simulink model "BikeModelDynWheels"  (R2017b)
settings: Solver=VariableStepAuto  StartTime=0.0  StopTime=10.0  RelTol=1e-3
undefined symbols (not defined in the file): b_contact, C_F_alpha, C_F_kappa, Cylinder, Dphi0, Dpsi0, epsilon, g, k_contact, lengthFF, lengthRF, lengthRW, locY, locZ, massRW, mB, mH, Parts_Lib, radiusRW, sigma, X, xPla, Y, yPla, Z, zPla
libraries: sm_lib x24, nesl_utility x18, vrlib x8, dspsrcs4 x1
(part 1 of 2)
settings Model: Creator=r_ahmed_afzal  LastModifiedBy=r_ahmed_afzal

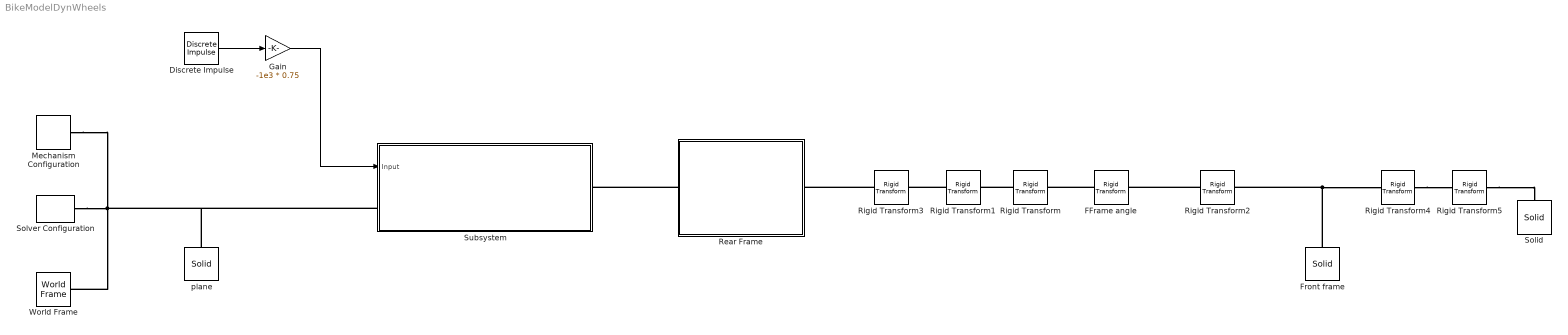
== system BikeModelDynWheels ==
  Discrete Impulse : dspsrcs4/Discrete  Impulse  Delay=0  SampleTime=1e-2  FrameSample=1  OutputFrames=off  dataType=double  isSigned=on  wordLen=16  udDataType=sfix(16)  fracBitsMode=Best precision  numFracBits=15  OutDataTypeStr=double  LastOutDataTypeStr=double
  FFrame angle : sm_lib/Frames and Transforms/Rigid Transform  TranslationMethod=None  TranslationStandardOffset=0  TranslationLengthUnit=m  TranslationStandardAxis=+Z  TranslationCartesianOffset=[0 0 0]  TranslationROffset=0  TranslationROffsetUnits=m  TranslationZOffset=0  TranslationZOffsetUnits=m  TranslationThetaOffset=0  TranslationThetaOffsetUnits=deg  RotationMethod=StandardAxis  RotationAngleUnits=rad  RotationStandardAxis=+X  RotationAngle=angleFF  RotationArbitraryAxis=[0 0 1]  FollAlignAxisA=+X  BaseAlignAxisA=+Y  FollAlignAxisB=+Y  BaseAlignAxisB=+Z  RotationSequenceAxes=FollowerAxes  RotationSequence=XYX  RotationSequenceAngles=[0 0 0]  RotationSequenceAnglesUnits=deg  RotationMatrix=[1 0 0; 0 1 0; 0 0 1]
  Front frame : sm_lib/Body Elements/Solid  InertiaType=Custom  Mass=mH  MassUnits=kg  CenterOfMass=[0 0 0]  CenterOfMassUnits=m  MomentsOfInertia=[1 1 1]  MomentsOfInertiaUnits=kg*m^2  ProductsOfInertia=[1 1 1]  ProductsOfInertiaUnits=kg*m^2  DensityBased=on  Density=1000  DensityUnits=kg/m^3  DoExposeReferenceFrame=on  SerializedFrames=<Frames/>  GraphicType=FromGeometry  MarkerShape=Sphere  MarkerSize=10  GraphicVisPropType=SimpleVisualProperties  GraphicDiffuseColor=[0.2 0.6 0.0]  GraphicSpecularColor=[0.5 0.5 0.5 1.0]  GraphicAmbientColor=[0.15 0.15 0.15 1.0]  GraphicEmissiveColor=[0.0 0.0 0.0 1.0]  GraphicShininess=75  GraphicOpacity=1.0  GeometryShape=Cylinder  RectangleSize=[1 1]  RectangleSizeUnits=m  BrickDimensions=[1 1 1]  BrickDimensionUnits=m  CylinderRadius=cylFF  CylinderRadiusUnits=m  CylinderLength=lengthFF  CylinderLengthUnits=m  SphereRadius=1  SphereRadiusUnits=m  EllipsoidRadii=[1 1 1]  EllipsoidRadiiUnits=m  ExtrusionCrossSection=[1 1; -1 1; -1 -1; 1 -1]  ExtrusionCrossSectionUnits=m  ExtrusionLength=1  ExtrusionLengthUnits=m  PolygonNumSides=3  PolygonOuterRadius=1  PolygonOuterRadiusUnits=m  ExtGeomFileType=STEP  ExtGeomFileUnits=m  RevolutionCrossSection=[1 1; 1 -1; 2 -1; 2 1]  RevolutionCrossSectionUnits=m  RevolutionExtent=Full  RevolutionAngle=180  RevolutionAngleUnits=deg
  Gain : Gain  Gain=-1e3 * 0.75
  Mechanism Configuration : sm_lib/Utilities/Mechanism Configuration  UniformGravity=Constant  GravityVector=[0 0 -g]  GravityUnits=m/s^2  LinearizationDelta=0.001
  Rear Frame : Subsystem
  Rigid Transform : sm_lib/Frames and Transforms/Rigid Transform  TranslationMethod=None  TranslationStandardOffset=0  TranslationLengthUnit=m  TranslationStandardAxis=+Z  TranslationCartesianOffset=[0 0 0]  TranslationROffset=0  TranslationROffsetUnits=m  TranslationZOffset=0  TranslationZOffsetUnits=m  TranslationThetaOffset=0  TranslationThetaOffsetUnits=deg  RotationMethod=None  RotationAngleUnits=deg  RotationStandardAxis=+Z  RotationAngle=0.0  RotationArbitraryAxis=[0 0 1]  FollAlignAxisA=+X  BaseAlignAxisA=+Y  FollAlignAxisB=+Y  BaseAlignAxisB=+Z  RotationSequenceAxes=FollowerAxes  RotationSequence=XYX  RotationSequenceAngles=[0 0 0]  RotationSequenceAnglesUnits=deg  RotationMatrix=[1 0 0; 0 1 0; 0 0 1]
  Rigid Transform1 : sm_lib/Frames and Transforms/Rigid Transform  TranslationMethod=None  TranslationStandardOffset=0  TranslationLengthUnit=m  TranslationStandardAxis=+Z  TranslationCartesianOffset=[0 0 0]  TranslationROffset=0  TranslationROffsetUnits=m  TranslationZOffset=0  TranslationZOffsetUnits=m  TranslationThetaOffset=0  TranslationThetaOffsetUnits=deg  RotationMethod=StandardAxis  RotationAngleUnits=rad  RotationStandardAxis=+X  RotationAngle=angleRF  RotationArbitraryAxis=[0 0 1]  FollAlignAxisA=+X  BaseAlignAxisA=+Y  FollAlignAxisB=+Y  BaseAlignAxisB=+Z  RotationSequenceAxes=FollowerAxes  RotationSequence=XYX  RotationSequenceAngles=[0 0 0]  RotationSequenceAnglesUnits=deg  RotationMatrix=[1 0 0; 0 1 0; 0 0 1]
  Rigid Transform2 : sm_lib/Frames and Transforms/Rigid Transform  TranslationMethod=StandardAxis  TranslationStandardOffset=lengthFF/2  TranslationLengthUnit=m  TranslationStandardAxis=+Z  TranslationCartesianOffset=[0 0 0]  TranslationROffset=0  TranslationROffsetUnits=m  TranslationZOffset=0  TranslationZOffsetUnits=m  TranslationThetaOffset=0  TranslationThetaOffsetUnits=deg  RotationMethod=None  RotationAngleUnits=deg  RotationStandardAxis=+Z  RotationAngle=0.0  RotationArbitraryAxis=[0 0 1]  FollAlignAxisA=+X  BaseAlignAxisA=+Y  FollAlignAxisB=+Y  BaseAlignAxisB=+Z  RotationSequenceAxes=FollowerAxes  RotationSequence=XYX  RotationSequenceAngles=[0 0 0]  RotationSequenceAnglesUnits=deg  RotationMatrix=[1 0 0; 0 1 0; 0 0 1]
  Rigid Transform3 : sm_lib/Frames and Transforms/Rigid Transform  TranslationMethod=StandardAxis  TranslationStandardOffset=lengthRF/2  TranslationLengthUnit=m  TranslationStandardAxis=+Z  TranslationCartesianOffset=[0 0 0]  TranslationROffset=0  TranslationROffsetUnits=m  TranslationZOffset=0  TranslationZOffsetUnits=m  TranslationThetaOffset=0  TranslationThetaOffsetUnits=deg  RotationMethod=None  RotationAngleUnits=deg  RotationStandardAxis=+Z  RotationAngle=0.0  RotationArbitraryAxis=[0 0 1]  FollAlignAxisA=+X  BaseAlignAxisA=+Y  FollAlignAxisB=+Y  BaseAlignAxisB=+Z  RotationSequenceAxes=FollowerAxes  RotationSequence=XYX  RotationSequenceAngles=[0 0 0]  RotationSequenceAnglesUnits=deg  RotationMatrix=[1 0 0; 0 1 0; 0 0 1]
  Rigid Transform4 : sm_lib/Frames and Transforms/Rigid Transform  TranslationMethod=StandardAxis  TranslationStandardOffset=lengthFF/2  TranslationLengthUnit=m  TranslationStandardAxis=+Z  TranslationCartesianOffset=[0 0 0]  TranslationROffset=0  TranslationROffsetUnits=m  TranslationZOffset=0  TranslationZOffsetUnits=m  TranslationThetaOffset=0  TranslationThetaOffsetUnits=deg  RotationMethod=StandardAxis  RotationAngleUnits=rad  RotationStandardAxis=-X  RotationAngle=angleFF  RotationArbitraryAxis=[0 0 1]  FollAlignAxisA=+X  BaseAlignAxisA=+Y  FollAlignAxisB=+Y  BaseAlignAxisB=+Z  RotationSequenceAxes=FollowerAxes  RotationSequence=XYX  RotationSequenceAngles=[0 0 0]  RotationSequenceAnglesUnits=deg  RotationMatrix=[1 0 0; 0 1 0; 0 0 1]
  Rigid Transform5 : sm_lib/Frames and Transforms/Rigid Transform  TranslationMethod=None  TranslationStandardOffset=0  TranslationLengthUnit=m  TranslationStandardAxis=+Z  TranslationCartesianOffset=[0 0 0]  TranslationROffset=0  TranslationROffsetUnits=m  TranslationZOffset=0  TranslationZOffsetUnits=m  TranslationThetaOffset=0  TranslationThetaOffsetUnits=deg  RotationMethod=AlignedAxes  RotationAngleUnits=deg  RotationStandardAxis=+Z  RotationAngle=0.0  RotationArbitraryAxis=[0 0 1]  FollAlignAxisA=+X  BaseAlignAxisA=+Z  FollAlignAxisB=+Z  BaseAlignAxisB=-X  RotationSequenceAxes=FollowerAxes  RotationSequence=XYX  RotationSequenceAngles=[0 0 0]  RotationSequenceAnglesUnits=deg  RotationMatrix=[1 0 0; 0 1 0; 0 0 1]
  Solid : sm_lib/Body Elements/Solid  InertiaType=CalculateFromGeometry  Mass=1  MassUnits=kg  CenterOfMass=[0 0 0]  CenterOfMassUnits=m  MomentsOfInertia=[1 1 1]  MomentsOfInertiaUnits=kg*m^2  ProductsOfInertia=[1 1 1]  ProductsOfInertiaUnits=kg*m^2  DensityBased=on  Density=1000  DensityUnits=kg/m^3  DoExposeReferenceFrame=on  SerializedFrames=<Frames/>  GraphicType=FromGeometry  MarkerShape=Sphere  MarkerSize=10  GraphicVisPropType=SimpleVisualProperties  GraphicDiffuseColor=[0.5 0.5 0.5]  GraphicSpecularColor=[0.5 0.5 0.5 1.0]  GraphicAmbientColor=[0.15 0.15 0.15 1.0]  GraphicEmissiveColor=[0.0 0.0 0.0 1.0]  GraphicShininess=75  GraphicOpacity=1.0  GeometryShape=Cylinder  RectangleSize=[1 1]  RectangleSizeUnits=m  BrickDimensions=[1 1 1]  BrickDimensionUnits=m  CylinderRadius=radiusFW  CylinderRadiusUnits=m  CylinderLength=lengthFW  CylinderLengthUnits=m  SphereRadius=1  SphereRadiusUnits=m  EllipsoidRadii=[1 1 1]  EllipsoidRadiiUnits=m  ExtrusionCrossSection=[1 1; -1 1; -1 -1; 1 -1]  ExtrusionCrossSectionUnits=m  ExtrusionLength=1  ExtrusionLengthUnits=m  PolygonNumSides=3  PolygonOuterRadius=1  PolygonOuterRadiusUnits=m  ExtGeomFileType=STEP  ExtGeomFileUnits=m  RevolutionCrossSection=[1 1; 1 -1; 2 -1; 2 1]  RevolutionCrossSectionUnits=m  RevolutionExtent=Full  RevolutionAngle=180  RevolutionAngleUnits=deg
  Solver Configuration : nesl_utility/Solver Configuration  PhysicalDomain=network_engine_domain  SubClassName=solver  LeftPortType=input  RightPortType=generic  Accelerate=off  Tones=[]  Harmonics=[]  SimulateNoise=off  Profile=off  UseLocalSampling=off  EnableSwitchedLinearOptims=on  FrequencyDomain=off  UseCCode=off  RelTol=0.001  AbsTol=1e-06  MinStep=1e-09  ToWorkspace=off  RevertToSquareIcSolve=off  NumHomotopyIterations=100  PhasorMode=off  PhasorModeNumHarmonics=1  DoDC=off  ResidualTolerance=1e-09  UseLocalSolver=off  LocalSolverChoice=NE_BACKWARD_EULER_ADVANCER  LocalSolverSampleTime=0.001  DoFixedCost=off  MaxNonlinIter=3  MaxModeIter=2  LinearAlgebra=Sparse  DelaysMemoryBudget=1024  AutomaticFiltering=on  FilteringTimeConstant=0.001
  Subsystem : Subsystem
  World Frame : sm_lib/Frames and Transforms/World Frame
  plane : sm_lib/Body Elements/Solid  InertiaType=CalculateFromGeometry  Mass=1  MassUnits=kg  CenterOfMass=[0 0 0]  CenterOfMassUnits=m  MomentsOfInertia=[1 1 1]  MomentsOfInertiaUnits=kg*m^2  ProductsOfInertia=[1 1 1]  ProductsOfInertiaUnits=kg*m^2  DensityBased=on  Density=1000  DensityUnits=kg/m^3  DoExposeReferenceFrame=on  SerializedFrames=<Frames/>  GraphicType=FromGeometry  MarkerShape=Sphere  MarkerSize=10  GraphicVisPropType=SimpleVisualProperties  GraphicDiffuseColor=[0.5 0.5 0.5]  GraphicSpecularColor=[0.5 0.5 0.5 1.0]  GraphicAmbientColor=[0.15 0.15 0.15 1.0]  GraphicEmissiveColor=[0.0 0.0 0.0 1.0]  GraphicShininess=75  GraphicOpacity=0.5  GeometryShape=Brick  RectangleSize=[1 1]  RectangleSizeUnits=m  BrickDimensions=[xPla yPla zPla]  BrickDimensionUnits=m  CylinderRadius=1  CylinderRadiusUnits=m  CylinderLength=1  CylinderLengthUnits=m  SphereRadius=1  SphereRadiusUnits=m  EllipsoidRadii=[1 1 1]  EllipsoidRadiiUnits=m  ExtrusionCrossSection=[1 1; -1 1; -1 -1; 1 -1]  ExtrusionCrossSectionUnits=m  ExtrusionLength=1  ExtrusionLengthUnits=m  PolygonNumSides=3  PolygonOuterRadius=1  PolygonOuterRadiusUnits=m  ExtGeomFileType=STEP  ExtGeomFileUnits=m  RevolutionCrossSection=[1 1; 1 -1; 2 -1; 2 1]  RevolutionCrossSectionUnits=m  RevolutionExtent=Full  RevolutionAngle=180  RevolutionAngleUnits=deg
  wires:
  Discrete Impulse/1 -> Gain/1
  Gain/1 -> Subsystem/1(Input)
  connections:
  Mechanism Configuration/RConn1 -- Subsystem/LConn1 -- plane/RConn1 -- Solver Configuration/RConn1 -- World Frame/RConn1
  Rear Frame/LConn1 -- Subsystem/RConn1
  Rigid Transform3/LConn1 -- Rear Frame/RConn1
  Rigid Transform1/LConn1 -- Rigid Transform3/RConn1
  Rigid Transform/LConn1 -- Rigid Transform1/RConn1
  FFrame angle/LConn1 -- Rigid Transform/RConn1
  Rigid Transform2/LConn1 -- FFrame angle/RConn1
  Front frame/RConn1 -- Rigid Transform4/LConn1 -- Rigid Transform2/RConn1
  Rigid Transform5/RConn1 -- Solid/RConn1
  Rigid Transform4/RConn1 -- Rigid Transform5/LConn1

== system BikeModelDynWheels/Rear Frame ==
  Rframe : sm_lib/Body Elements/Solid  InertiaType=Custom  Mass=mB  MassUnits=kg  CenterOfMass=[0 locY locZ]  CenterOfMassUnits=m  MomentsOfInertia=[1 1 1]  MomentsOfInertiaUnits=kg*m^2  ProductsOfInertia=[1 1 1]  ProductsOfInertiaUnits=kg*m^2  DensityBased=on  Density=1000  DensityUnits=kg/m^3  DoExposeReferenceFrame=on  SerializedFrames=<Frames/>  GraphicType=FromGeometry  MarkerShape=Sphere  MarkerSize=10  GraphicVisPropType=SimpleVisualProperties  GraphicDiffuseColor=[0.2 0.6 0.0]  GraphicSpecularColor=[0.5 0.5 0.5 1.0]  GraphicAmbientColor=[0.15 0.15 0.15 1.0]  GraphicEmissiveColor=[0.0 0.0 0.0 1.0]  GraphicShininess=75  GraphicOpacity=1.0  GeometryShape=Cylinder  RectangleSize=[1 1]  RectangleSizeUnits=m  BrickDimensions=[1 1 1]  BrickDimensionUnits=m  CylinderRadius=cylRF  CylinderRadiusUnits=m  CylinderLength=lengthRF  CylinderLengthUnits=m  SphereRadius=1  SphereRadiusUnits=m  EllipsoidRadii=[1 1 1]  EllipsoidRadiiUnits=m  ExtrusionCrossSection=[1 1; -1 1; -1 -1; 1 -1]  ExtrusionCrossSectionUnits=m  ExtrusionLength=1  ExtrusionLengthUnits=m  PolygonNumSides=3  PolygonOuterRadius=1  PolygonOuterRadiusUnits=m  ExtGeomFileType=STEP  ExtGeomFileUnits=m  RevolutionCrossSection=[1 1; 1 -1; 2 -1; 2 1]  RevolutionCrossSectionUnits=m  RevolutionExtent=Full  RevolutionAngle=180  RevolutionAngleUnits=deg
  Rigid Transform : sm_lib/Frames and Transforms/Rigid Transform  TranslationMethod=None  TranslationStandardOffset=0  TranslationLengthUnit=m  TranslationStandardAxis=+Z  TranslationCartesianOffset=[0 0 0]  TranslationROffset=0  TranslationROffsetUnits=m  TranslationZOffset=0  TranslationZOffsetUnits=m  TranslationThetaOffset=0  TranslationThetaOffsetUnits=deg  RotationMethod=StandardAxis  RotationAngleUnits=deg  RotationStandardAxis=+Y  RotationAngle=90  RotationArbitraryAxis=[0 0 1]  FollAlignAxisA=+X  BaseAlignAxisA=+Y  FollAlignAxisB=+Y  BaseAlignAxisB=+Z  RotationSequenceAxes=FollowerAxes  RotationSequence=XYX  RotationSequenceAngles=[0 0 0]  RotationSequenceAnglesUnits=deg  RotationMatrix=[1 0 0; 0 1 0; 0 0 1]
  Rigid Transform1 : sm_lib/Frames and Transforms/Rigid Transform  TranslationMethod=None  TranslationStandardOffset=0  TranslationLengthUnit=m  TranslationStandardAxis=+Z  TranslationCartesianOffset=[0 0 0]  TranslationROffset=0  TranslationROffsetUnits=m  TranslationZOffset=0  TranslationZOffsetUnits=m  TranslationThetaOffset=0  TranslationThetaOffsetUnits=deg  RotationMethod=StandardAxis  RotationAngleUnits=rad  RotationStandardAxis=-X  RotationAngle=angleRF  RotationArbitraryAxis=[0 0 1]  FollAlignAxisA=+X  BaseAlignAxisA=+Y  FollAlignAxisB=+Y  BaseAlignAxisB=+Z  RotationSequenceAxes=FollowerAxes  RotationSequence=XYX  RotationSequenceAngles=[0 0 0]  RotationSequenceAnglesUnits=deg  RotationMatrix=[1 0 0; 0 1 0; 0 0 1]
  Rigid Transform2 : sm_lib/Frames and Transforms/Rigid Transform  TranslationMethod=StandardAxis  TranslationStandardOffset=lengthRF/2  TranslationLengthUnit=m  TranslationStandardAxis=+Z  TranslationCartesianOffset=[0 0 0]  TranslationROffset=0  TranslationROffsetUnits=m  TranslationZOffset=0  TranslationZOffsetUnits=m  TranslationThetaOffset=0  TranslationThetaOffsetUnits=deg  RotationMethod=None  RotationAngleUnits=deg  RotationStandardAxis=+Z  RotationAngle=0.0  RotationArbitraryAxis=[0 0 1]  FollAlignAxisA=+X  BaseAlignAxisA=+Y  FollAlignAxisB=+Y  BaseAlignAxisB=+Z  RotationSequenceAxes=FollowerAxes  RotationSequence=XYX  RotationSequenceAngles=[0 0 0]  RotationSequenceAnglesUnits=deg  RotationMatrix=[1 0 0; 0 1 0; 0 0 1]
  Conn1 : PMIOPort  Port=1  Side=Left
  Conn2 : PMIOPort  Port=2  Side=Right
  connections:
  Rigid Transform1/LConn1 -- Rigid Transform/RConn1
  Rframe/RConn1 -- Conn2/RConn1 -- Rigid Transform2/RConn1
  Rigid Transform/LConn1 -- Conn1/RConn1
  Rigid Transform2/LConn1 -- Rigid Transform1/RConn1

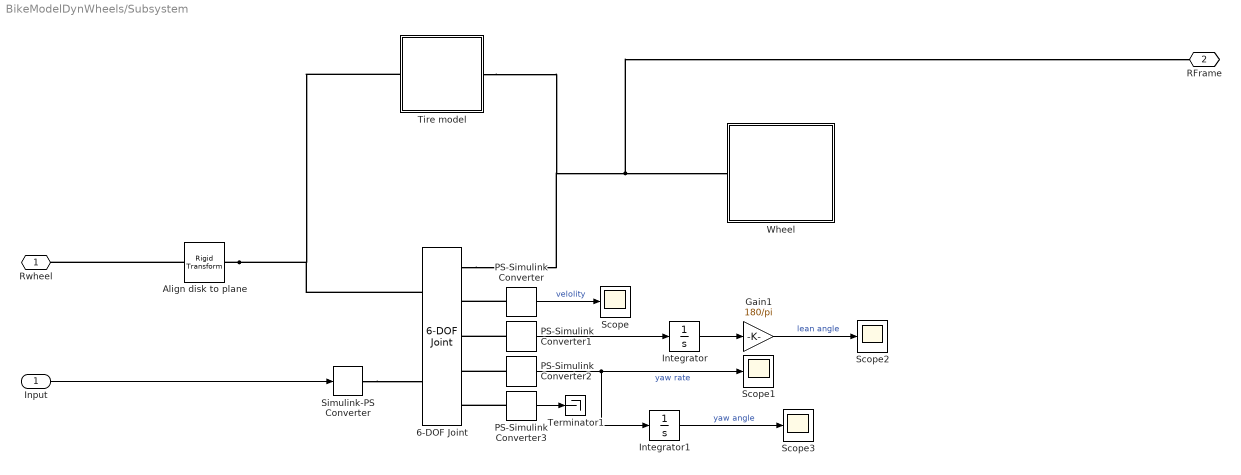
== system BikeModelDynWheels/Subsystem ==
  Input : Inport
  6-DOF Joint : sm_lib/Joints/6-DOF Joint  SenseConstraintForce=off  SenseConstraintForceX=off  SenseConstraintForceY=off  SenseConstraintForceZ=off  SenseConstraintTorque=off  SenseConstraintTorqueX=off  SenseConstraintTorqueY=off  SenseConstraintTorqueZ=off  SenseTotalForce=off  SenseTotalForceX=off  SenseTotalForceY=off  SenseTotalForceZ=off  SenseTotalTorque=off  SenseTotalTorqueX=off  SenseTotalTorqueY=off  SenseTotalTorqueZ=off  CompositeWrenchDir=FollowerOnBase  CompositeWrenchFrame=BaseFrame  PxEquilibriumPosition=0  PxEquilibriumPositionUnits=m  PxSpringStiffness=0  PxSpringStiffnessUnits=N/m  PxDampingCoefficient=0  PxDampingCoefficientUnits=N/(m/s)  PxTorqueActuationMode=NoTorque  PxMotionActuationMode=ComputedMotion  PxSensePosition=off  PxSenseVelocity=on  PxSenseAcceleration=off  PxSenseTorqueForce=off  PxPositionTargetSpecify=on  PxPositionTargetPriority=High  PxPositionTargetValue=-xPla/2 + 0.1  PxPositionTargetValueUnits=m  PxVelocityTargetSpecify=off  PxVelocityTargetPriority=High  PxVelocityTargetValue=v0  PxVelocityTargetValueUnits=m/s  PyEquilibriumPosition=0  PyEquilibriumPositionUnits=m  PySpringStiffness=0  PySpringStiffnessUnits=N/m  PyDampingCoefficient=0  PyDampingCoefficientUnits=N/(m/s)  PyTorqueActuationMode=NoTorque  PyMotionActuationMode=ComputedMotion  PySensePosition=off  PySenseVelocity=off  PySenseAcceleration=off  PySenseTorqueForce=off  PyPositionTargetSpecify=on  PyPositionTargetPriority=High  PyPositionTargetValue=radiusRW  PyPositionTargetValueUnits=m  PyVelocityTargetSpecify=off  PyVelocityTargetPriority=High  PyVelocityTargetValue=0  PyVelocityTargetValueUnits=m/s  PzEquilibriumPosition=0  PzEquilibriumPositionUnits=m  PzSpringStiffness=0  PzSpringStiffnessUnits=N/m  PzDampingCoefficient=0  PzDampingCoefficientUnits=N/(m/s)  PzTorqueActuationMode=NoTorque  PzMotionActuationMode=ComputedMotion  PzSensePosition=off  PzSenseVelocity=off  PzSenseAcceleration=off  PzSenseTorqueForce=off  PzPositionTargetSpecify=off  PzPositionTargetPriority=High  PzPositionTargetValue=0  PzPositionTargetValueUnits=m  PzVelocityTargetSpecify=off  PzVelocityTargetPriority=High  PzVelocityTargetValue=0  PzVelocityTargetValueUnits=m/s  SphDefPosRotationMethod=None  SphDefPosRotationAngleUnits=deg  SphDefPosRotationStandardAxis=+Z  SphDefPosRotationAngle=0.0  SphDefPosRotationArbitraryAxis=[0 0 1]  SphDefPosFollAlignAxisA=+X  SphDefPosBaseAlignAxisA=+Y  SphDefPosFollAlignAxisB=+Y  SphDefPosBaseAlignAxisB=+Z  SphDefPosRotationSequenceAxes=FollowerAxes  SphDefPosRotationSequence=XYX  SphDefPosRotationSequenceAngles=[0 0 0]  SphDefPosRotationSequenceAnglesUnits=deg  SphDefPosRotationMatrix=[1 0 0; 0 1 0; 0 0 1]  SphEqPosRotationMethod=None  SphEqPosRotationAngleUnits=deg  SphEqPosRotationStandardAxis=+Z  SphEqPosRotationAngle=0.0  SphEqPosRotationArbitraryAxis=[0 0 1]  SphEqPosFollAlignAxisA=+X  SphEqPosBaseAlignAxisA=+Y  SphEqPosFollAlignAxisB=+Y  SphEqPosBaseAlignAxisB=+Z  SphEqPosRotationSequenceAxes=FollowerAxes  SphEqPosRotationSequence=XYX  SphEqPosRotationSequenceAngles=[0 0 0]  SphEqPosRotationSequenceAnglesUnits=deg  SphEqPosRotationMatrix=[1 0 0; 0 1 0; 0 0 1]  SphSpringStiffness=0  SphSpringStiffnessUnits=N*m/deg  SphDampingCoefficient=0  SphDampingCoefficientUnits=N*m/(deg/s)  SphActuateTorqueX=off  SphActuateTorqueY=off  SphActuateTorqueZ=on  SphActuateTorque=off  SphTorqueActuationMode=InputTorque  SphMotionActuationMode=ComputedMotion  SphActuationFrame=FollowerFrame  SphSensePosition=off  SphSenseVelocityX=on  SphSenseVelocityY=on  SphSenseVelocityZ=on  SphSenseVelocity=off  SphSenseAccelerationX=off  SphSenseAccelerationY=off  SphSenseAccelerationZ=off  SphSenseAcceleration=off  SphSenseTorqueX=off  SphSenseTorqueY=off  SphSenseTorqueZ=off  SphSenseTorqueForce=off  SphSensingFrame=FollowerFrame  SphPositionTargetRotationMethod=StandardAxis  SphPositionTargetRotationAngleUnits=deg  SphPositionTargetRotationStandardAxis=+X  SphPositionTargetRotationAngle=phi0  SphPositionTargetRotationArbitraryAxis=[0 0 1]  SphPositionTargetFollAlignAxisA=+X  SphPositionTargetBaseAlignAxisA=+Y  SphPositionTargetFollAlignAxisB=+Y  SphPositionTargetBaseAlignAxisB=+Z  SphPositionTargetRotationSequenceAxes=FollowerAxes  SphPositionTargetRotationSequence=XYX  SphPositionTargetRotationSequenceAngles=[0 0 0]  SphPositionTargetRotationSequenceAnglesUnits=deg  SphPositionTargetRotationMatrix=[1 0 0; 0 1 0; 0 0 1]  SphPositionTargetSpecify=off  SphPositionTargetPriority=High  SphVelocityTargetValue=[Dphi0 Dpsi0 0]  SphVelocityTargetValueUnits=rad/s  SphVelocityTargetSpecify=on  SphVelocityTargetPriority=High  SphVelocityTargetInFollowerFrame=on
  Align disk to plane : sm_lib/Frames and Transforms/Rigid Transform  TranslationMethod=None  TranslationStandardOffset=0  TranslationLengthUnit=m  TranslationStandardAxis=+Z  TranslationCartesianOffset=[0 0 0]  TranslationROffset=0  TranslationROffsetUnits=m  TranslationZOffset=0  TranslationZOffsetUnits=m  TranslationThetaOffset=0  TranslationThetaOffsetUnits=deg  RotationMethod=AlignedAxes  RotationAngleUnits=deg  RotationStandardAxis=-X  RotationAngle=90  RotationArbitraryAxis=[0 0 1]  FollAlignAxisA=+Y  BaseAlignAxisA=+Z  FollAlignAxisB=+X  BaseAlignAxisB=+X  RotationSequenceAxes=FollowerAxes  RotationSequence=XYX  RotationSequenceAngles=[0 0 0]  RotationSequenceAnglesUnits=deg  RotationMatrix=[1 0 0; 0 1 0; 0 0 1]
  Gain1 : Gain  Gain=180/pi
  Integrator : Integrator
  Integrator1 : Integrator
  PS-Simulink Converter{,1..3} (4 alike) : nesl_utility/PS-Simulink Converter  PhysicalDomain=network_engine_domain  SubClassName=ps_output  LeftPortType=input  RightPortType=output  PseudoPeriodic=off  Frequencies=[]  Unit=1  AffineConversion=off
  Scope{,1..3} (4 alike) : Scope
  Simulink-PS Converter : nesl_utility/Simulink-PS Converter  PhysicalDomain=network_engine_domain  SubClassName=ps_input  LeftPortType=input  RightPortType=output  PseudoPeriodic=off  Frequencies=[]  NoiseDistribution=none  NoiseParameters=[]  Unit=1  AffineConversion=off  FilteringAndDerivatives=provide  SimscapeFilterOrder=1  InputFilterTimeConstant=0.001  UdotUserProvided=0
  Terminator1 : Terminator
  Tire model : Subsystem
  Wheel : Subsystem  Tag=CustomStyle  AncestorBlock=Parts_Lib/Cylinder  mask(Solid Cylinder with Markings){cyl_radius=radiusRW, cyl_length=lengthRW, cyl_density=1000, cyl_color=blue, cyl_opacity=1, cyl_color_custom=[0.7920    0.9900    0.9900], mark_radius=[0.75 0.5], mark_len_factor=1.01, mark_angle=60, mark_color=purple, mark_opacity=1}
      mask prompts: cyl_radius "Radius (m)"; cyl_length "Length (m)"; cyl_density "Density (kg/m^3)"; cyl_color "Color"; cyl_opacity "Opacity (0-1)"; cyl_color_custom "Custom Color (rgb)"; mark_radius "Outer, inner radius (% of cylinder radius)"; mark_len_factor "Length (factor of cylinder length)"; mark_angle "Sweep angle (deg)"; mark_color "Color"; mark_opacity "Opacity (0-1)"
      mask init:
      | curblk = gcb;
      | if strcmp(get_param(curblk,'cyl_color'),'red')
      |     set_param([curblk '/Cylinder'],'GraphicDiffuseColor','[0.8 0.0 0.2]');
      |     set_param(curblk,'BackGroundColor','[0.901961, 0.396078, 0.396078]');
      | elseif strcmp(get_param(gcb,'cyl_color'),'blue')
      |     set_param([curblk '/Cylinder'],'GraphicDiffuseColor','[0.0 0.5 0.7]');
      |     set_param(curblk,'BackGroundColor','[0.541176, 0.698039, 0.901961]');
      | elseif strcmp(get_param(gcb,'cyl_color'),'yellow')
      |     set_param([curblk '/Cylinder'],'GraphicDiffuseColor','[1.0 1.0 0.0]');
      |     set_param(curblk,'BackGroundColor','[0.905882, 0.890196, 0.392157]');
      | elseif strcmp(get_param(gcb,'cyl_color'),'gray')
      |     set_param([curblk '/Cylinder'],'GraphicDiffuseColor','[1.0 1.0 1.0]*0.6');
      |     set_param(curblk,'BackGroundColor','[0.6 0.6 0.6]');
      | elseif strcmp(get_param(gcb,'cyl_color'),'custom')
      |     set_param([curblk '/Cylinder'],'GraphicDiffuseColor',get_param(curblk,'cyl_color_custom'));
      |     set_param(curblk,'BackGroundColor','[1 1 1]');
      | end
      | 
      | if strcmp(get_param(curblk,'mark_color'),'purple')
      |     set_param([curblk '/Vis1'],'GraphicDiffuseColor','[0.4 0.0 0.4]');
      |     set_param([curblk '/Vis2'],'GraphicDiffuseColor','[0.4 0.0 0.4]');
      | elseif strcmp(get_param(gcb,'mark_color'),'green')
      |     set_param([curblk '/Vis1'],'GraphicDiffuseColor','[0.0 0.8 0.0]');
      |     set_param([curblk '/Vis2'],'GraphicDiffuseColor','[0.0 0.8 0.0]');
      | elseif strcmp(get_param(gcb,'mark_color'),'orange')
      |     set_param([curblk '/Vis1'],'GraphicDiffuseColor','[1.0 0.6 0.0]');
      |     set_param([curblk '/Vis2'],'GraphicDiffuseColor','[1.0 0.6 0.0]');
      | elseif strcmp(get_param(gcb,'mark_color'),'black')
      |     set_param([curblk '/Vis1'],'GraphicDiffuseColor','[0.0 0.0 0.0]');
      |     set_param([curblk '/Vis2'],'GraphicDiffuseColor','[0.0 0.0 0.0]');
      | end
      | 
      | clear curblk
      mask TypeOptions cyl_color: red | gray | yellow | blue | custom
      mask Callback cyl_color:
      | maskObj = Simulink.Mask.get(gcb);
      | clr_h = maskObj.getParameter('cyl_color_custom');
      | if strcmp(get_param(gcb,'cyl_color'),'custom')
      |     clr_h.Visible = 'on';
      | else
      |     clr_h.Visible = 'off';
      | end
      mask TypeOptions mark_color: purple | green | orange | black
      mask DialogControl Container4 Prompt: Cylinder
      mask DialogControl Container7 Prompt: Markings
  Rwheel : PMIOPort  Port=1  Side=Left
  RFrame : PMIOPort  Port=2  Side=Right
  wires:
  PS-Simulink Converter/1 -> Scope/1  "velolity"
  Input/1 -> Simulink-PS Converter/1
  Integrator/1 -> Gain1/1
  Gain1/1 -> Scope2/1  "lean angle"
  PS-Simulink Converter2/1 -> Integrator1/1, Scope1/1  "yaw rate"
  PS-Simulink Converter3/1 -> Terminator1/1
  Integrator1/1 -> Scope3/1  "yaw angle"
  PS-Simulink Converter1/1 -> Integrator/1
  connections:
  Align disk to plane/LConn1 -- Rwheel/RConn1
  PS-Simulink Converter3/LConn1 -- 6-DOF Joint/RConn5
  Simulink-PS Converter/RConn1 -- 6-DOF Joint/LConn2
  PS-Simulink Converter2/LConn1 -- 6-DOF Joint/RConn4
  PS-Simulink Converter/LConn1 -- 6-DOF Joint/RConn2
  PS-Simulink Converter1/LConn1 -- 6-DOF Joint/RConn3
  Align disk to plane/RConn1 -- 6-DOF Joint/LConn1 -- Tire model/LConn1
  6-DOF Joint/RConn1 -- Tire model/RConn1 -- RFrame/RConn1 -- Wheel/LConn1

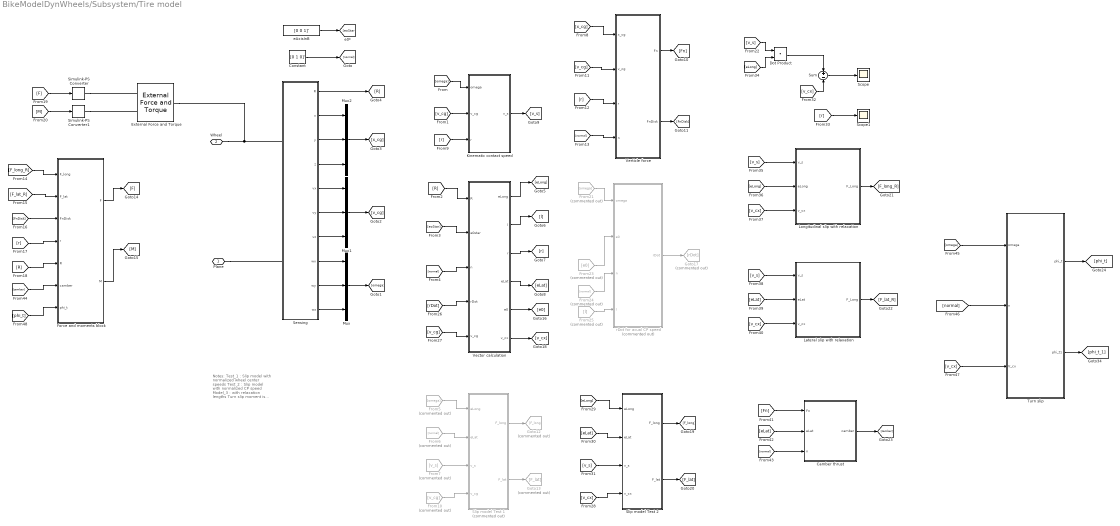
== system BikeModelDynWheels/Subsystem/Tire model ==
  note: Notes:
      | Test_1 : Slip model with normalized wheel center speeds
      | Test_2 : Slip model with normalized CP speed
      | Model_3 : with relaxation lengths
      |
      | Turn slip moment is excluded in the model as per the
      | paper by RS Sharp
  Camber thrust : Subsystem
  Constant : Constant  Value=[0 1 0]'
  Dot Product : DotProduct  InputSameDT=on  OutDataTypeStr=Inherit: Inherit via internal rule
  External Force and Torque : sm_lib/Forces and Torques/External Force and Torque  ForceResolutionFrame=AttachedFrame  EnableForceX=off  EnableForceY=off  EnableForceZ=off  EnableForce=on  TorqueResolutionFrame=AttachedFrame  EnableTorqueX=off  EnableTorqueY=off  EnableTorqueZ=off  EnableTorque=on
  Force and moments block : Subsystem
  From10 : From  Commented=on  GotoTag=v_cg
  From21 : From  Commented=on  GotoTag=omega
  From23 : From  Commented=on  GotoTag=e0
  From24 : From  Commented=on  GotoTag=normal
  From25 : From  Commented=on  GotoTag=l
  From5 : From  Commented=on  GotoTag=omega
  From6 : From  Commented=on  GotoTag=normal
  From7 : From  Commented=on  GotoTag=v_s
  Goto12 : Goto  Commented=on  GotoTag=F_long
  Goto13 : Goto  Commented=on  GotoTag=F_lat
  Goto17 : Goto  Commented=on  GotoTag=rDot
  Kinematic contact speed : Subsystem
  Lateral slip with relaxation : Subsystem
  Longitudinal slip with relaxation : Subsystem
  Mux : Mux  Inputs=3
  Mux1 : Mux  Inputs=3
  Mux2 : Mux  Inputs=3
  Scope : Scope
  Scope1 : Scope
  Sensing : Subsystem
  Simulink-PS Converter : nesl_utility/Simulink-PS Converter  PhysicalDomain=network_engine_domain  SubClassName=ps_input  LeftPortType=input  RightPortType=output  PseudoPeriodic=off  Frequencies=[]  NoiseDistribution=none  NoiseParameters=[]  Unit=1  AffineConversion=off  FilteringAndDerivatives=provide  SimscapeFilterOrder=1  InputFilterTimeConstant=0.001  UdotUserProvided=0
  Simulink-PS Converter1 : nesl_utility/Simulink-PS Converter  PhysicalDomain=network_engine_domain  SubClassName=ps_input  LeftPortType=input  RightPortType=output  PseudoPeriodic=off  Frequencies=[]  NoiseDistribution=none  NoiseParameters=[]  Unit=1  AffineConversion=off  FilteringAndDerivatives=provide  SimscapeFilterOrder=1  InputFilterTimeConstant=0.001  UdotUserProvided=0
  Slip model Test 1 : Subsystem  Commented=on
  Slip model Test 2 : Subsystem
  Sum : Sum  Inputs=+-
  Turn slip : Subsystem
  Vector calculation : Subsystem
  Verticle force : Subsystem
  eAxisInB : Constant  Value=[0 0 1]'
  rDot for acual CP speed : Subsystem  Commented=on
  Plane : PMIOPort  Port=1  Side=Left
  Wheel : PMIOPort  Port=2  Side=Right
  wires:
  eAxisInB/1 -> [eoStar]
  Constant/1 -> [normal]
  Sensing/8(wx) -> Mux/1
  Sensing/9(wy) -> Mux/2
  Sensing/10(wz) -> Mux/3
  Mux/1 -> [omega]
  [omega] -> Kinematic contact speed/1(omega)
  Sensing/5(vx) -> Mux1/1
  Sensing/6(vy) -> Mux1/2
  Sensing/7(vz) -> Mux1/3
  Mux1/1 -> [v_cg]
  [v_cg] -> Kinematic contact speed/2(v_cg)
  Sensing/2(x) -> Mux2/1
  Sensing/3(y) -> Mux2/2
  Sensing/4(z) -> Mux2/3
  Mux2/1 -> [x_cg]
  Sensing/1(R) -> [R]
  [R] -> Vector calculation/1(R)
  [eoStar] -> Vector calculation/2(e0star)
  [normal] -> Vector calculation/3(n)
  From5/1 -> Slip model Test 1/1(eLong)
  From6/1 -> Slip model Test 1/2(eLat)
  Vector calculation/1(eLong) -> [eLong]
  Vector calculation/2(l) -> [l]
  Vector calculation/3(r) -> [r]
  Vector calculation/4(eLat) -> [eLat]
  [r] -> Kinematic contact speed/3(r)
  Kinematic contact speed/1(v_s) -> [v_s]
  From7/1 -> Slip model Test 1/3(v_s)
  From10/1 -> Slip model Test 1/4(v_cg)
  [x_cg] -> Verticle force/1(x_cg)
  [v_cg] -> Verticle force/2(v_cg)
  [r] -> Verticle force/3(r)
  [normal] -> Verticle force/4(n)
  Verticle force/1(Fn) -> [Fn]
  Verticle force/2(FnDisk) -> [FnDisk]
  Slip model Test 1/1(F_long) -> Goto12/1
  Slip model Test 1/2(F_lat) -> Goto13/1
  [F_long_R] -> Force and moments block/1(F_long)
  [F_lat_R] -> Force and moments block/2(F_lat)
  [FnDisk] -> Force and moments block/3(FnDisk)
  [r] -> Force and moments block/4(r)
  [R] -> Force and moments block/5(R)
  Force and moments block/1(F) -> [F]
  Force and moments block/2(M) -> [M]
  [F] -> Simulink-PS Converter/1
  [M] -> Simulink-PS Converter1/1
  From21/1 -> rDot for acual CP speed/1(omega)
  Vector calculation/5(e0) -> [e0]
  From23/1 -> rDot for acual CP speed/2(e0)
  From24/1 -> rDot for acual CP speed/3(n)
  From25/1 -> rDot for acual CP speed/4(l)
  rDot for acual CP speed/1(rDot) -> Goto17/1
  [rDot] -> Vector calculation/4(rDot)
  [v_cg] -> Vector calculation/5(v_cg)
  Vector calculation/6(v_cx) -> [v_cx]
  Slip model Test 2/1(F_long) -> [F_long]
  [v_s] -> Slip model Test 2/3(v_s)
  [eLat] -> Slip model Test 2/2(eLat)
  [eLong] -> Slip model Test 2/1(eLong)
  Slip model Test 2/2(F_lat) -> [F_lat]
  [v_cx] -> Slip model Test 2/4(v_cx)
  [v_cx] -> Sum/2
  Sum/1 -> Scope/1
  [r] -> Scope1/1
  [v_s] -> Dot Product/1
  [eLong] -> Dot Product/2
  Dot Product/1 -> Sum/1
  [v_s] -> Longitudinal slip with relaxation/1(v_s)
  [eLong] -> Longitudinal slip with relaxation/2(eLong)
  [v_cx] -> Longitudinal slip with relaxation/3(v_cx)
  Longitudinal slip with relaxation/1(F_Long) -> [F_long_R]
  [eLat] -> Lateral slip with relaxation/2(eLat)
  Lateral slip with relaxation/1(F_Long) -> [F_lat_R]
  [v_cx] -> Lateral slip with relaxation/3(v_cx)
  [v_s] -> Lateral slip with relaxation/1(v_s)
  [Fn] -> Camber thrust/1(Fn)
  [eLat] -> Camber thrust/2(eLat)
  [normal] -> Camber thrust/3(n)
  Camber thrust/1(camber) -> [camber]
  Turn slip/1(phi_t) -> [phi_t]
  [v_cx] -> Turn slip/3(V_cx)
  Turn slip/2(phi_t1) -> [phi_t_1]
  [omega] -> Turn slip/1(omega)
  [normal] -> Turn slip/2(n)
  [camber] -> Force and moments block/6(camber)
  [phi_t] -> Force and moments block/7(phi_t)
  connections:
  Plane/RConn1 -- Sensing/LConn2
  Wheel/RConn1 -- External Force and Torque/RConn1 -- Sensing/LConn1
  Simulink-PS Converter/RConn1 -- External Force and Torque/LConn1
  Simulink-PS Converter1/RConn1 -- External Force and Torque/LConn2

== system BikeModelDynWheels/Subsystem/Wheel ==
  Cylinder : sm_lib/Body Elements/Solid  InertiaType=Custom  Mass=massRW  MassUnits=kg  CenterOfMass=[0 0 0]  CenterOfMassUnits=m  MomentsOfInertia=momentInertiaRW  MomentsOfInertiaUnits=kg*m^2  ProductsOfInertia=[0 0 0]  ProductsOfInertiaUnits=kg*m^2  DensityBased=on  Density=cyl_density  DensityUnits=kg/(m^3)  DoExposeReferenceFrame=on  SerializedFrames=<Frames/>  GraphicType=FromGeometry  MarkerShape=Sphere  MarkerSize=10  MarkerSizeUnits=m  GraphicVisPropType=SimpleVisualProperties  GraphicDiffuseColor=[0.0 0.5 0.7]  GraphicSpecularColor=[0.5 0.5 0.5 1.0]  GraphicAmbientColor=[0.15 0.15 0.15 1.0]  GraphicEmissiveColor=[0.0 0.0 0.0 1.0]  GraphicShininess=75  GraphicOpacity=cyl_opacity  GeometryShape=Cylinder  RectangleSize=[1 1]  RectangleSizeUnits=m  BrickDimensions=[1 1 1]  BrickDimensionUnits=m  CylinderRadius=cyl_radius  CylinderRadiusUnits=m  CylinderLength=cyl_length  CylinderLengthUnits=m  SphereRadius=1  SphereRadiusUnits=m  EllipsoidRadii=[1 1 1]  EllipsoidRadiiUnits=m  ExtrusionCrossSection=[1 1; -1 1; -1 -1; 1 -1]  ExtrusionCrossSectionUnits=m  ExtrusionLength=1  ExtrusionLengthUnits=m  PolygonNumSides=3  PolygonOuterRadius=1  PolygonOuterRadiusUnits=m  ExtGeomFileType=STL  ExtGeomFileUnits=m  RevolutionCrossSection=[1 1; 1 -1; 2 -1; 2 1]  RevolutionCrossSectionUnits=m  RevolutionExtent=Full  RevolutionAngle=180  RevolutionAngleUnits=deg
  Transform Vis2 : sm_lib/Frames and Transforms/Rigid Transform  TranslationMethod=None  TranslationStandardOffset=0  TranslationLengthUnit=m  TranslationStandardAxis=+Z  TranslationCartesianOffset=[0 0 0]  TranslationROffset=0  TranslationROffsetUnits=m  TranslationZOffset=0  TranslationZOffsetUnits=m  TranslationThetaOffset=0  TranslationThetaOffsetUnits=deg  RotationMethod=StandardAxis  RotationAngleUnits=deg  RotationStandardAxis=+Y  RotationAngle=180  RotationArbitraryAxis=[0 0 1]  FollAlignAxisA=+X  BaseAlignAxisA=+Y  FollAlignAxisB=+Y  BaseAlignAxisB=+Z  RotationSequenceAxes=FollowerAxes  RotationSequence=XYX  RotationSequenceAngles=[0 0 0]  RotationSequenceAnglesUnits=deg  RotationMatrix=[1 0 0; 0 1 0; 0 0 1]
  Vis1 : sm_lib/Body Elements/Solid  InertiaType=CalculateFromGeometry  Mass=1  MassUnits=kg  CenterOfMass=[0 0 0]  CenterOfMassUnits=m  MomentsOfInertia=[1 1 1]  MomentsOfInertiaUnits=kg*m^2  ProductsOfInertia=[0 0 0]  ProductsOfInertiaUnits=kg*m^2  DensityBased=on  Density=1e-3  DensityUnits=kg/(m^3)  DoExposeReferenceFrame=on  SerializedFrames=<Frames/>  GraphicType=FromGeometry  MarkerShape=Sphere  MarkerSize=10  MarkerSizeUnits=m  GraphicVisPropType=SimpleVisualProperties  GraphicDiffuseColor=[0.4 0.0 0.4]  GraphicSpecularColor=[0.5 0.5 0.5 1.0]  GraphicAmbientColor=[0.15 0.15 0.15 1.0]  GraphicEmissiveColor=[0.0 0.0 0.0 1.0]  GraphicShininess=75  GraphicOpacity=mark_opacity  GeometryShape=GeneralSolidOfRevolution  RectangleSize=[1 1]  RectangleSizeUnits=m  BrickDimensions=[1 1 1]  BrickDimensionUnits=m  CylinderRadius=0.1  CylinderRadiusUnits=m  CylinderLength=0.01  CylinderLengthUnits=m  SphereRadius=1  SphereRadiusUnits=m  EllipsoidRadii=[1 1 1]  EllipsoidRadiiUnits=m  ExtrusionCrossSection=[1 1; -1 1; -1 -1; 1 -1]  ExtrusionCrossSectionUnits=m  ExtrusionLength=1  ExtrusionLengthUnits=m  PolygonNumSides=3  PolygonOuterRadius=1  PolygonOuterRadiusUnits=m  ExtGeomFileType=STL  ExtGeomFileUnits=m  RevolutionCrossSection=[cyl_radius*mark_radius(1) cyl_length/2*mark_len_factor; cyl_radius*mark_radius(2) cyl_length/2*mark_len_factor; cyl_radius*mark_radius(2) -cyl_length/2*mark_len_factor; cyl_radius*mark_radius(1) -cyl_length/2*mark_len_factor]  RevolutionCrossSectionUnits=m  RevolutionExtent=Custom  RevolutionAngle=mark_angle  RevolutionAngleUnits=deg
  Vis2 : sm_lib/Body Elements/Solid  InertiaType=CalculateFromGeometry  Mass=1  MassUnits=kg  CenterOfMass=[0 0 0]  CenterOfMassUnits=m  MomentsOfInertia=[1 1 1]  MomentsOfInertiaUnits=kg*m^2  ProductsOfInertia=[0 0 0]  ProductsOfInertiaUnits=kg*m^2  DensityBased=on  Density=1e-3  DensityUnits=kg/(m^3)  DoExposeReferenceFrame=on  SerializedFrames=<Frames/>  GraphicType=FromGeometry  MarkerShape=Sphere  MarkerSize=10  MarkerSizeUnits=m  GraphicVisPropType=SimpleVisualProperties  GraphicDiffuseColor=[0.4 0.0 0.4]  GraphicSpecularColor=[0.5 0.5 0.5 1.0]  GraphicAmbientColor=[0.15 0.15 0.15 1.0]  GraphicEmissiveColor=[0.0 0.0 0.0 1.0]  GraphicShininess=75  GraphicOpacity=mark_opacity  GeometryShape=GeneralSolidOfRevolution  RectangleSize=[1 1]  RectangleSizeUnits=m  BrickDimensions=[1 1 1]  BrickDimensionUnits=m  CylinderRadius=0.1  CylinderRadiusUnits=m  CylinderLength=0.01  CylinderLengthUnits=m  SphereRadius=1  SphereRadiusUnits=m  EllipsoidRadii=[1 1 1]  EllipsoidRadiiUnits=m  ExtrusionCrossSection=[1 1; -1 1; -1 -1; 1 -1]  ExtrusionCrossSectionUnits=m  ExtrusionLength=1  ExtrusionLengthUnits=m  PolygonNumSides=3  PolygonOuterRadius=1  PolygonOuterRadiusUnits=m  ExtGeomFileType=STL  ExtGeomFileUnits=m  RevolutionCrossSection=[cyl_radius*mark_radius(1) cyl_length/2*mark_len_factor; cyl_radius*mark_radius(2) cyl_length/2*mark_len_factor; cyl_radius*mark_radius(2) -cyl_length/2*mark_len_factor; cyl_radius*mark_radius(1) -cyl_length/2*mark_len_factor]  RevolutionCrossSectionUnits=m  RevolutionExtent=Custom  RevolutionAngle=mark_angle  RevolutionAngleUnits=deg
  R : PMIOPort  Port=1  Side=Left
  connections:
  Vis2/RConn1 -- Transform Vis2/RConn1
  Vis1/RConn1 -- Transform Vis2/LConn1 -- Cylinder/RConn1 -- R/RConn1

== system BikeModelDynWheels/Subsystem/Tire model/Camber thrust ==
  Fn : Inport
  eLat : Inport  Port=2
  n : Inport  Port=3
  Dot Product : DotProduct  InputSameDT=on  OutDataTypeStr=Inherit: Inherit via internal rule
  Product : Product
  Product1 : Product
  camber : Outport
  wires:
  Dot Product/1 -> Product/2  "sin_gamma"
  Fn/1 -> Product/1
  Product/1 -> Product1/1
  Product1/1 -> camber/1
  n/1 -> Dot Product/1
  eLat/1 -> Product1/2, Dot Product/2

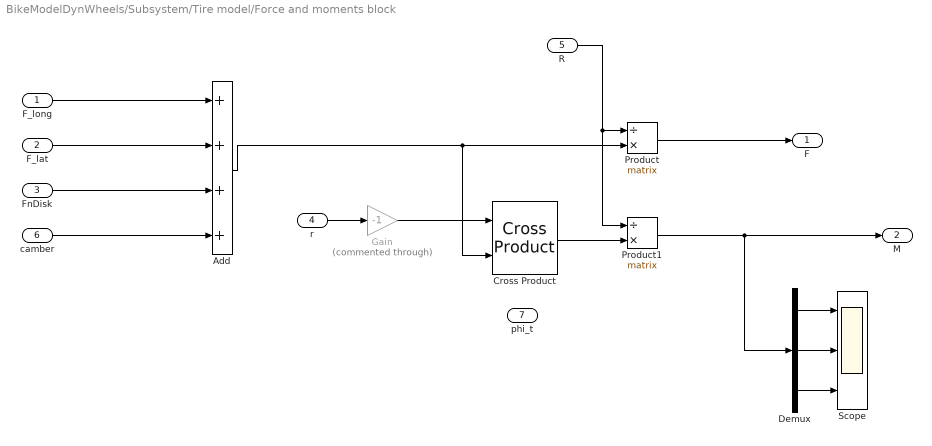
== system BikeModelDynWheels/Subsystem/Tire model/Force and moments block ==
  F_long : Inport
  F_lat : Inport  Port=2
  FnDisk : Inport  Port=3
  r : Inport  Port=4
  R : Inport  Port=5
  camber : Inport  Port=6
  phi_t : Inport  Port=7
  Add : Sum  Inputs=4
  Cross Product : vrlib/Utilities/Cross Product
      settings: SourceProductBaseCode=VR
  Demux : Demux  Outputs=3
  Gain : Gain  Commented=through  Gain=-1
  Product : Product  Inputs=/*  Multiplication=Matrix(*)
  Product1 : Product  Inputs=/*  Multiplication=Matrix(*)
  Scope : Scope  NumInputPorts=3
  F : Outport
  M : Outport  Port=2
  wires:
  FnDisk/1 -> Add/3
  Add/1 -> Cross Product/2, Product/2
  Product/1 -> F/1
  R/1 -> Product1/1, Product/1
  r/1 -> Gain/1
  Product1/1 -> Demux/1, M/1
  Gain/1 -> Cross Product/1
  F_long/1 -> Add/1
  F_lat/1 -> Add/2
  Demux/3 -> Scope/3
  Demux/2 -> Scope/2
  Demux/1 -> Scope/1
  camber/1 -> Add/4
  Cross Product/1 -> Product1/2

== system BikeModelDynWheels/Subsystem/Tire model/Kinematic contact speed ==
  omega : Inport
  v_cg : Inport  Port=2
  r : Inport  Port=3
  Add : Sum
  Cross Product : vrlib/Utilities/Cross Product
      settings: SourceProductBaseCode=VR
  v_s : Outport
  wires:
  omega/1 -> Cross Product/1
  Cross Product/1 -> Add/2
  r/1 -> Cross Product/2
  v_cg/1 -> Add/1
  Add/1 -> v_s/1

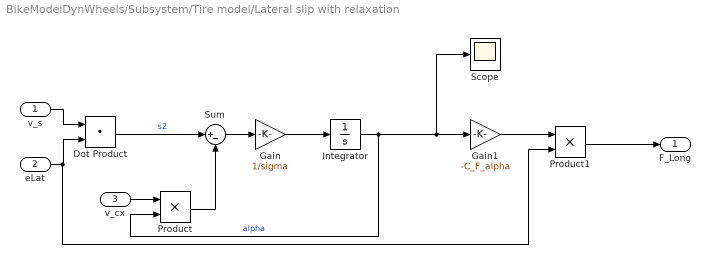
== system BikeModelDynWheels/Subsystem/Tire model/Lateral slip with relaxation ==
  v_s : Inport
  eLat : Inport  Port=2
  v_cx : Inport  Port=3
  Dot Product : DotProduct  InputSameDT=on  OutDataTypeStr=Inherit: Inherit via internal rule
  Gain : Gain  Gain=1/sigma
  Gain1 : Gain  Gain=-C_F_alpha
  Integrator : Integrator
  Product : Product
  Product1 : Product
  Scope : Scope
  Sum : Sum  Inputs=|+-
  F_Long : Outport
  wires:
  v_s/1 -> Dot Product/1
  eLat/1 -> Product1/2, Dot Product/2
  Dot Product/1 -> Sum/1  "s2"
  v_cx/1 -> Product/1
  Product/1 -> Sum/2
  Sum/1 -> Gain/1
  Gain/1 -> Integrator/1
  Integrator/1 -> Scope/1, Gain1/1, Product/2  "alpha"
  Gain1/1 -> Product1/1
  Product1/1 -> F_Long/1

== system BikeModelDynWheels/Subsystem/Tire model/Longitudinal slip with relaxation ==
  v_s : Inport
  eLong : Inport  Port=2
  v_cx : Inport  Port=3
  Dot Product : DotProduct  InputSameDT=on  OutDataTypeStr=Inherit: Inherit via internal rule
  Gain : Gain  Gain=1/sigma
  Gain1 : Gain  Gain=-C_F_kappa
  Integrator : Integrator
  Product : Product
  Product1 : Product
  Scope : Scope
  Sum : Sum  Inputs=|+-
  F_Long : Outport
  wires:
  v_s/1 -> Dot Product/1
  eLong/1 -> Product1/2, Dot Product/2
  Dot Product/1 -> Sum/1  "s1"
  v_cx/1 -> Product/1
  Product/1 -> Sum/2
  Sum/1 -> Gain/1
  Gain/1 -> Integrator/1
  Integrator/1 -> Scope/1, Gain1/1, Product/2  "kappa"
  Gain1/1 -> Product1/1
  Product1/1 -> F_Long/1

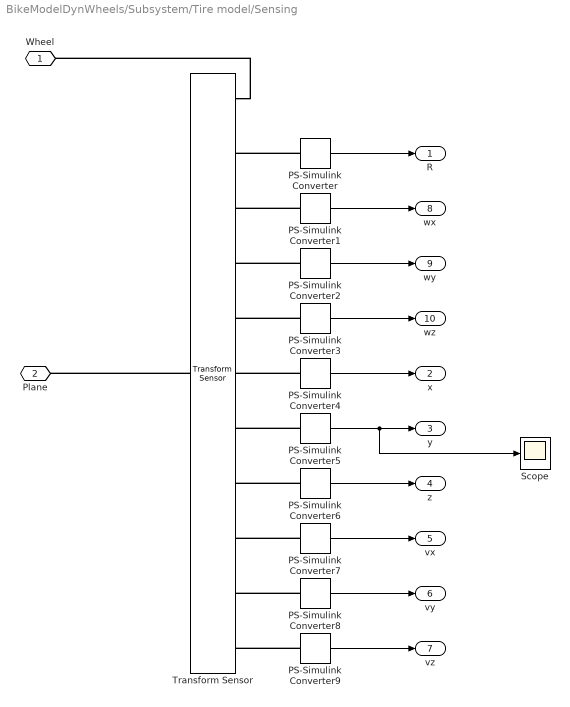
== system BikeModelDynWheels/Subsystem/Tire model/Sensing ==
  PS-Simulink Converter{,1..9} (10 alike) : nesl_utility/PS-Simulink Converter  PhysicalDomain=network_engine_domain  SubClassName=ps_output  LeftPortType=input  RightPortType=output  PseudoPeriodic=off  Frequencies=[]  Unit=1  AffineConversion=off
  Scope : Scope
  Transform Sensor : sm_lib/Frames and Transforms/Transform Sensor  MeasurementFrame=Base  SenseAngle=off  SenseAxis=off  SenseAngle1=off  SenseAngle2=off  SenseAngle3=off  SenseQ=off  SenseR=on  SenseOmegaX=on  SenseOmegaY=on  SenseOmegaZ=on  SenseOmega1=off  SenseOmega2=off  SenseOmega3=off  SenseQDot=off  SenseRDot=off  SenseAlphaX=off  SenseAlphaY=off  SenseAlphaZ=off  SenseAlpha1=off  SenseAlpha2=off  SenseAlpha3=off  SenseQDDot=off  SenseRDDot=off  SenseX=on  SenseY=on  SenseZ=on  SenseRad=off  SenseAzim=off  SenseDist=off  SenseInc=off  SenseXDot=on  SenseYDot=on  SenseZDot=on  SenseRadDot=off  SenseAzimDot=off  SenseDistDot=off  SenseIncDot=off  SenseXDDot=off  SenseYDDot=off  SenseZDDot=off  SenseRadDDot=off  SenseAzimDDot=off  SenseDistDDot=off  SenseIncDDot=off
  Wheel : PMIOPort  Port=1  Side=Left
  Plane : PMIOPort  Port=2  Side=Left
  R : Outport
  x : Outport  Port=2
  y : Outport  Port=3
  z : Outport  Port=4
  vx : Outport  Port=5
  vy : Outport  Port=6
  vz : Outport  Port=7
  wx : Outport  Port=8
  wy : Outport  Port=9
  wz : Outport  Port=10
  wires:
  PS-Simulink Converter2/1 -> wy/1
  PS-Simulink Converter8/1 -> vy/1
  PS-Simulink Converter9/1 -> vz/1
  PS-Simulink Converter1/1 -> wx/1
  PS-Simulink Converter4/1 -> x/1
  PS-Simulink Converter7/1 -> vx/1
  PS-Simulink Converter3/1 -> wz/1
  PS-Simulink Converter5/1 -> Scope/1, y/1
  PS-Simulink Converter6/1 -> z/1
  PS-Simulink Converter/1 -> R/1
  connections:
  PS-Simulink Converter1/LConn1 -- Transform Sensor/RConn3
  PS-Simulink Converter4/LConn1 -- Transform Sensor/RConn6
  PS-Simulink Converter3/LConn1 -- Transform Sensor/RConn5
  PS-Simulink Converter9/LConn1 -- Transform Sensor/RConn11
  PS-Simulink Converter2/LConn1 -- Transform Sensor/RConn4
  PS-Simulink Converter6/LConn1 -- Transform Sensor/RConn8
  PS-Simulink Converter/LConn1 -- Transform Sensor/RConn2
  Transform Sensor/LConn1 -- Plane/RConn1
  Transform Sensor/RConn1 -- Wheel/RConn1
  PS-Simulink Converter5/LConn1 -- Transform Sensor/RConn7
  PS-Simulink Converter7/LConn1 -- Transform Sensor/RConn9
  PS-Simulink Converter8/LConn1 -- Transform Sensor/RConn10

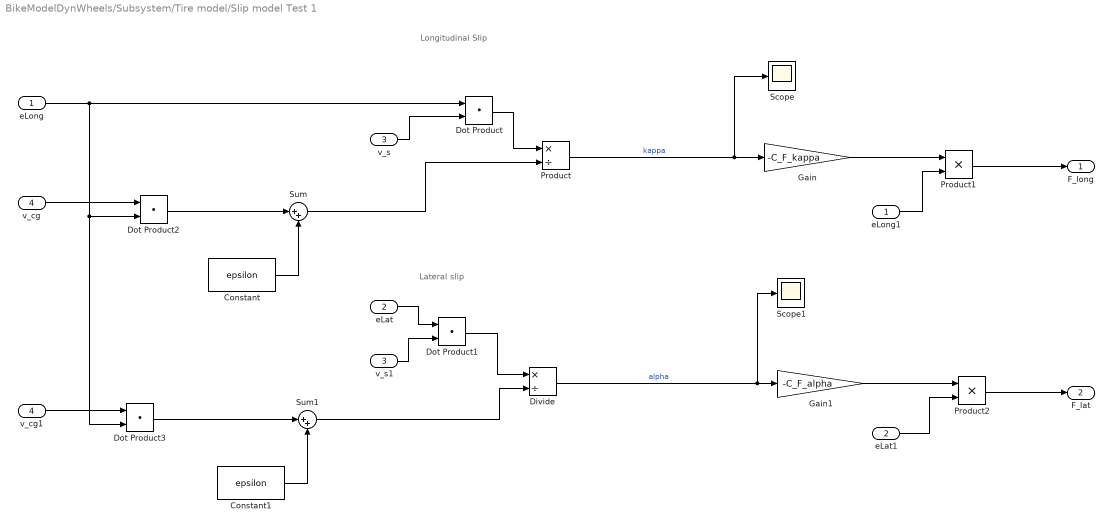
== system BikeModelDynWheels/Subsystem/Tire model/Slip model Test 1 ==
  note: Lateral slip
  note: Longitudinal Slip
  eLong : Inport
  eLat : Inport  Port=2
  v_s : Inport  Port=3
  v_cg : Inport  Port=4
  Constant : Constant  Value=epsilon
  Constant1 : Constant  Value=epsilon
  Divide : Product  Inputs=*/
  Dot Product{,1..3} (4 alike) : DotProduct  InputSameDT=on  OutDataTypeStr=Inherit: Inherit via internal rule
  Gain : Gain  Gain=-C_F_kappa
  Gain1 : Gain  Gain=-C_F_alpha
  Product : Product  Inputs=*/
  Product1 : Product
  Product2 : Product
  Scope : Scope
  Scope1 : Scope
  Sum : Sum  Inputs=|++
  Sum1 : Sum  Inputs=|++
  eLat1 : InportShadow  Port=2
  eLong1 : InportShadow
  v_cg1 : InportShadow  Port=4
  v_s1 : InportShadow  Port=3
  F_long : Outport
  F_lat : Outport  Port=2
  wires:
  eLong/1 -> Dot Product3/2, Dot Product2/2, Dot Product/1
  v_s/1 -> Dot Product/2
  Dot Product/1 -> Product/1
  Product/1 -> Scope/1, Gain/1  "kappa"
  eLat/1 -> Dot Product1/1
  v_s1/1 -> Dot Product1/2
  Dot Product1/1 -> Divide/1
  Divide/1 -> Scope1/1, Gain1/1  "alpha"
  Gain/1 -> Product1/1
  eLong1/1 -> Product1/2
  Gain1/1 -> Product2/1
  eLat1/1 -> Product2/2
  Product1/1 -> F_long/1
  Product2/1 -> F_lat/1
  Constant/1 -> Sum/2
  Sum/1 -> Product/2
  Constant1/1 -> Sum1/2
  Sum1/1 -> Divide/2
  v_cg/1 -> Dot Product2/1
  Dot Product2/1 -> Sum/1
  v_cg1/1 -> Dot Product3/1
  Dot Product3/1 -> Sum1/1

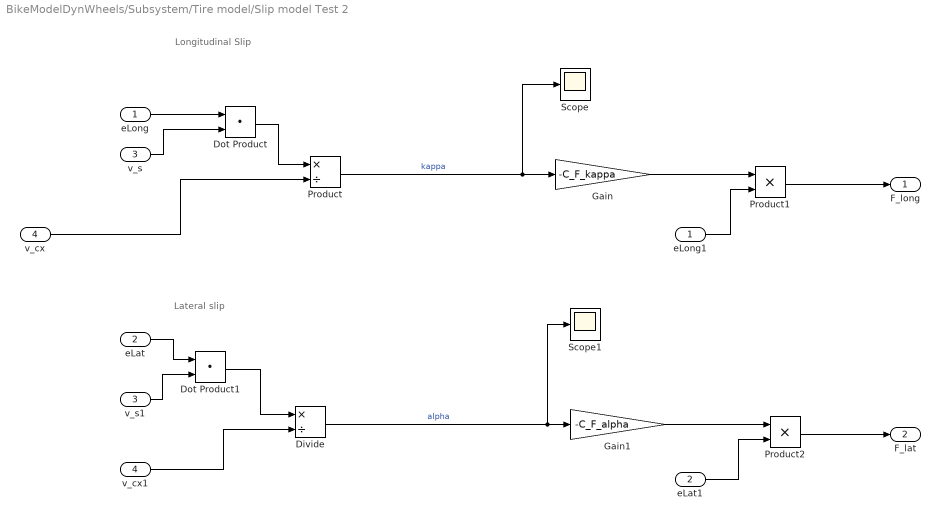
== system BikeModelDynWheels/Subsystem/Tire model/Slip model Test 2 ==
  note: Lateral slip
  note: Longitudinal Slip
  eLong : Inport
  eLat : Inport  Port=2
  v_s : Inport  Port=3
  v_cx : Inport  Port=4
  Divide : Product  Inputs=*/
  Dot Product : DotProduct  InputSameDT=on  OutDataTypeStr=Inherit: Inherit via internal rule
  Dot Product1 : DotProduct  InputSameDT=on  OutDataTypeStr=Inherit: Inherit via internal rule
  Gain : Gain  Gain=-C_F_kappa
  Gain1 : Gain  Gain=-C_F_alpha
  Product : Product  Inputs=*/
  Product1 : Product
  Product2 : Product
  Scope : Scope
  Scope1 : Scope
  eLat1 : InportShadow  Port=2
  eLong1 : InportShadow
  v_cx1 : InportShadow  Port=4
  v_s1 : InportShadow  Port=3
  F_long : Outport
  F_lat : Outport  Port=2
  wires:
  eLong/1 -> Dot Product/1
  v_s/1 -> Dot Product/2
  Dot Product/1 -> Product/1
  Product/1 -> Scope/1, Gain/1  "kappa"
  eLat/1 -> Dot Product1/1
  v_s1/1 -> Dot Product1/2
  Dot Product1/1 -> Divide/1
  Divide/1 -> Scope1/1, Gain1/1  "alpha"
  Gain/1 -> Product1/1
  eLong1/1 -> Product1/2
  Gain1/1 -> Product2/1
  eLat1/1 -> Product2/2
  Product1/1 -> F_long/1
  Product2/1 -> F_lat/1
  v_cx/1 -> Product/2
  v_cx1/1 -> Divide/2

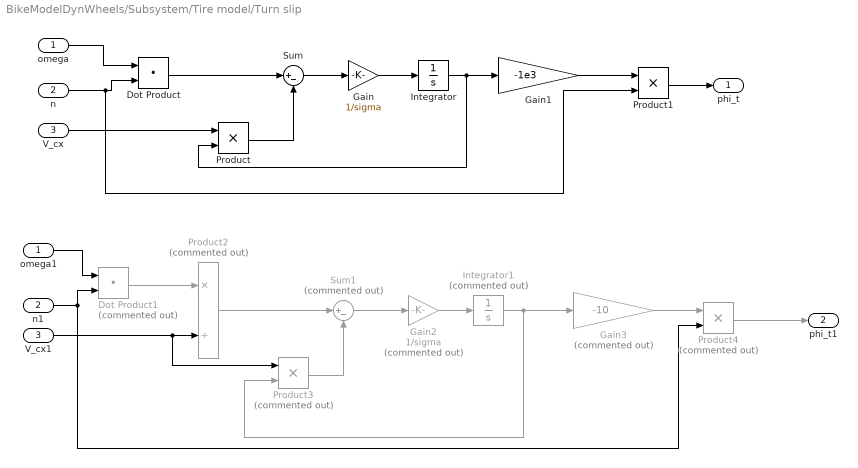
== system BikeModelDynWheels/Subsystem/Tire model/Turn slip ==
  omega : Inport
  n : Inport  Port=2
  V_cx : Inport  Port=3
  Dot Product : DotProduct  InputSameDT=on  OutDataTypeStr=Inherit: Inherit via internal rule
  Dot Product1 : DotProduct  Commented=on  InputSameDT=on  OutDataTypeStr=Inherit: Inherit via internal rule
  Gain : Gain  Gain=1/sigma
  Gain1 : Gain  Gain=-1e3
  Gain2 : Gain  Commented=on  Gain=1/sigma
  Gain3 : Gain  Commented=on  Gain=-10
  Integrator : Integrator
  Integrator1 : Integrator  Commented=on
  Product : Product
  Product1 : Product
  Product2 : Product  Commented=on  Inputs=*/
  Product3 : Product  Commented=on
  Product4 : Product  Commented=on
  Sum : Sum  Inputs=|+-
  Sum1 : Sum  Commented=on  Inputs=|+-
  V_cx1 : InportShadow  Port=3
  n1 : InportShadow  Port=2
  omega1 : InportShadow
  phi_t : Outport
  phi_t1 : Outport  Port=2
  wires:
  omega/1 -> Dot Product/1
  n/1 -> Product1/2, Dot Product/2
  Dot Product/1 -> Sum/1
  Sum/1 -> Gain/1
  Gain/1 -> Integrator/1
  Integrator/1 -> Product/2, Gain1/1
  Gain1/1 -> Product1/1
  Product1/1 -> phi_t/1
  Product/1 -> Sum/2
  V_cx/1 -> Product/1
  omega1/1 -> Dot Product1/1
  n1/1 -> Product4/2, Dot Product1/2
  Dot Product1/1 -> Product2/1
  V_cx1/1 -> Product3/1, Product2/2
  Product2/1 -> Sum1/1
  Sum1/1 -> Gain2/1
  Product3/1 -> Sum1/2
  Gain2/1 -> Integrator1/1
  Integrator1/1 -> Gain3/1, Product3/2
  Gain3/1 -> Product4/1
  Product4/1 -> phi_t1/1

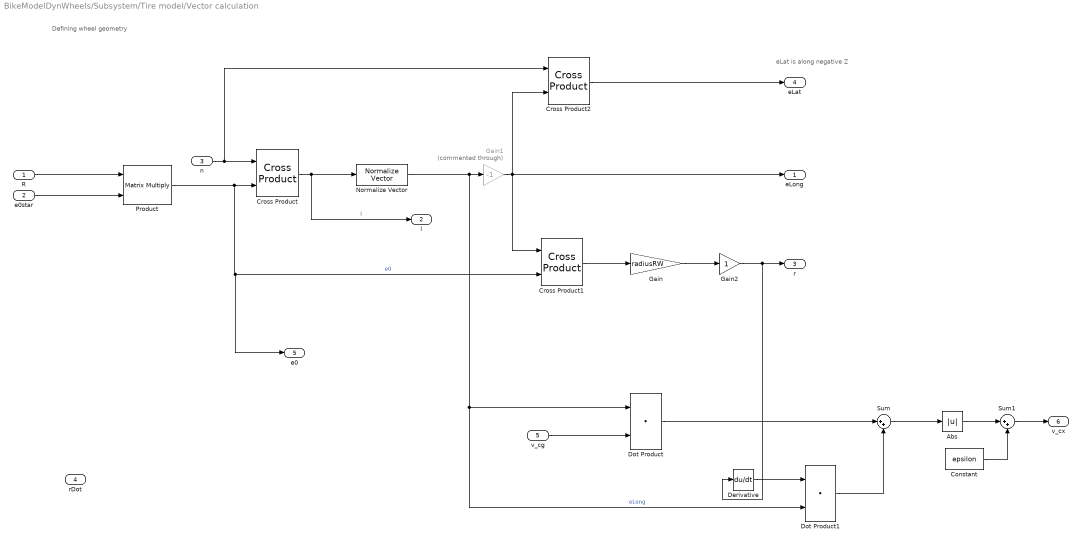
== system BikeModelDynWheels/Subsystem/Tire model/Vector calculation ==
  note: Defining wheel geometry
  note: eLat is along
      | negative Z
  R : Inport
  e0star : Inport  Port=2
  n : Inport  Port=3
  rDot : Inport  Port=4
  v_cg : Inport  Port=5
  Abs : Abs  ZeroCross=off
  Constant : Constant  Value=epsilon
  Cross Product : vrlib/Utilities/Cross Product
      settings: SourceProductBaseCode=VR
  Cross Product1 : vrlib/Utilities/Cross Product
      settings: SourceProductBaseCode=VR
  Cross Product2 : vrlib/Utilities/Cross Product
      settings: SourceProductBaseCode=VR
  Derivative : Derivative
  Dot Product : DotProduct  InputSameDT=on  OutDataTypeStr=Inherit: Inherit via internal rule
  Dot Product1 : DotProduct  InputSameDT=on  OutDataTypeStr=Inherit: Inherit via internal rule
  Gain : Gain  Gain=radiusRW
  Gain1 : Gain  Commented=through  Gain=-1
  Gain2 : Gain
  Normalize Vector : vrlib/Utilities/Normalize Vector  maxzero=0
      settings: SourceProductName=Simulink 3D Animation  SourceProductBaseCode=VR
  Product : Product  Multiplication=Matrix(*)
  Sum : Sum  Inputs=|++
  Sum1 : Sum  Inputs=|++
  eLong : Outport
  l : Outport  Port=2
  r : Outport  Port=3
  eLat : Outport  Port=4
  e0 : Outport  Port=5
  v_cx : Outport  Port=6
  wires:
  R/1 -> Product/1
  e0star/1 -> Product/2
  Product/1 -> Cross Product1/2, e0/1, Cross Product/2  "e0"
  n/1 -> Cross Product2/1, Cross Product/1
  Cross Product/1 -> l/1, Normalize Vector/1  "l"
  Normalize Vector/1 -> Dot Product/1, Dot Product1/2, Gain1/1  "eLong"
  Cross Product1/1 -> Gain/1
  Gain/1 -> Gain2/1
  Cross Product2/1 -> eLat/1
  v_cg/1 -> Dot Product/2
  Dot Product/1 -> Sum/1
  Sum/1 -> Abs/1
  Abs/1 -> Sum1/1
  Constant/1 -> Sum1/2
  Sum1/1 -> v_cx/1
  Gain1/1 -> eLong/1, Cross Product2/2, Cross Product1/1
  Derivative/1 -> Dot Product1/1
  Dot Product1/1 -> Sum/2
  Gain2/1 -> Derivative/1, r/1
